simulink model "example_2_slx"  (R2021b)
settings: Solver=VariableStepAuto  StartTime=0.0  StopTime=10.0  RelTol=1e-3
settings Model: Creator=yingguang wang  LastModifiedBy=yingguang wang
settings DataIOCC: InspectSignalLogs=on

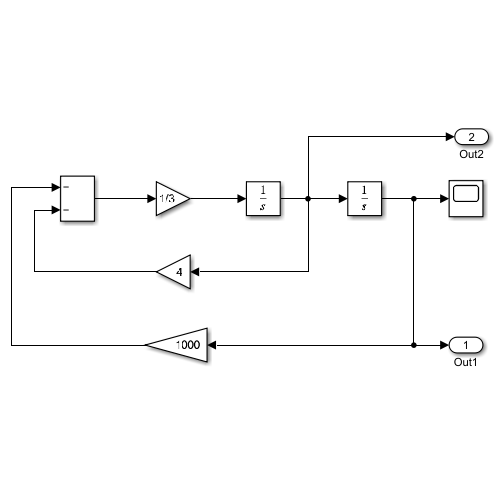
[thumbnail: Simulink's stored preview of the top-level diagram]
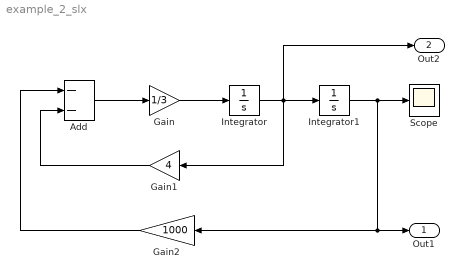
== system example_2_slx ==
  Add : Sum  Inputs=--
  Gain : Gain  Gain=1/3
  Gain1 : Gain  Gain=4
  Gain2 : Gain  Gain=1000
  Integrator : Integrator  InitialCondition=1
  Integrator1 : Integrator  InitialCondition=1
  Scope : Scope
  Out1 : Outport
  Out2 : Outport  Port=2
  wires:
  Add/1 -> Gain/1
  Gain/1 -> Integrator/1
  Integrator/1 -> Out2/1, Gain1/1, Integrator1/1
  Integrator1/1 -> Out1/1, Gain2/1, Scope/1
  Gain1/1 -> Add/2
  Gain2/1 -> Add/1
